simulink model "Host_IO_DataCapture"  (R2019b)
settings: Solver=FixedStepAuto  StartTime=0.0  StopTime=inf  FixedStep=(1/fpga_clk_rate)*4096  RelTol=1e-3  EnableMultiTasking=on
InitFcn:
  | model_init
values from neighbouring files (symbols this model uses):
  end_inc = round (((f1*2^N)/fpga_clk_rate)/VectorSamplingFactor)    [model_init.m]
  fpga_clk_rate = Fs/VectorSamplingFactor    (= 128000000)    [model_init.m]
  frameSize = 1536    [model_init.m]
  LFM_counter_inc = round((end_inc-start_inc)/PulseWidth_count)    [model_init.m]
  PulseWidth_count = pspshared.libiio.aximm.write(                    'IPAddress',IPAddr,                    'AddressOffset',hex2dec('13C'))    [SimplePulseGenerator_4x4_HDL_IQ_IIO_script.m]    (also in model_init.m = 640)
  RangeDelayTrigger_count = pspshared.libiio.aximm.write(                    'IPAddress',IPAddr,                    'AddressOffset',hex2dec('138'))    [SimplePulseGenerator_4x4_HDL_IQ_IIO_script.m]    (also in model_init.m = 1)
  start_inc = round (((f0*2^N)/fpga_clk_rate)/VectorSamplingFactor)    [model_init.m]
libraries: hdlsllib x16, simulink x2, psp_axi_iio_lib x1
Description:
  | 4x4 IQ ADC/DAC Data capture model for host PC
  | 
  | This model demonstrates capturing data from the FPGA for IQ mixer data. AXI4 register is used
  | to switch between different ADC channels and collect frames of data at every
  | time step of the simulation
  | 
  | The DAC is driven by an NCO. It's frequency is also adjustable from this model as well.
settings Model: Creator=darenlee  LastModifiedBy=ajtro
settings SolverCC: PositivePriorityOrder=on
settings DataIOCC: ReturnWorkspaceOutputs=off
settings OptimizationCC: DefaultParameterBehavior=Inlined  EnhancedBackFolding=on  PassReuseOutputArgsAs=Individual arguments  MaxStackSize=64  OptimizeBlockOrder=speed  DifferentSizesBufferReuse=on  OptimizationCustomize=off  EfficientTunableParamExpr=on
settings DebuggingCC: ParameterTunabilityLossMsg=error  PregeneratedLibrarySubsystemCodeDiagnostic=none  ArithmeticOperatorsInVariantConditions=warning
settings HardwareCC: ProdBitPerPointer=32  ProdBitPerSizeT=32  ProdBitPerPtrDiffT=32  ProdLargestAtomicInteger=Long  ProdLargestAtomicFloat=Double  ProdWordSize=32  ProdLongLongMode=on  ProdHWDeviceType=ARM Compatible->ARM Cortex
settings SFSimCC: SimUseLocalCustomCode=off  MATLABDynamicMemAlloc=off  CustomCodeUndefinedFunction=UseInterfaceOnly
settings RTWCC: SystemTargetFile=ert.tlc  TemplateMakefile=ert_default_tmf  GenerateReport=on  RTWUseLocalCustomCode=off  Toolchain=Linaro AArch32 Linux v6.3.1  IncludeHyperlinkInReport=on  LaunchReport=on  GenerateTraceInfo=on  GenerateTraceReport=on  GenerateTraceReportSl=on  GenerateTraceReportSf=on  GenerateTraceReportEml=on
settings CodeAppCC: ForceParamTrailComments=on  IgnoreCustomStorageClasses=off  OperatorAnnotations=on  SimulinkDataObjDesc=on  SFDataObjDesc=on  InsertBlockDesc=on
settings ERTTargetCC: ERTCustomFileTemplate=example_file_process.tlc

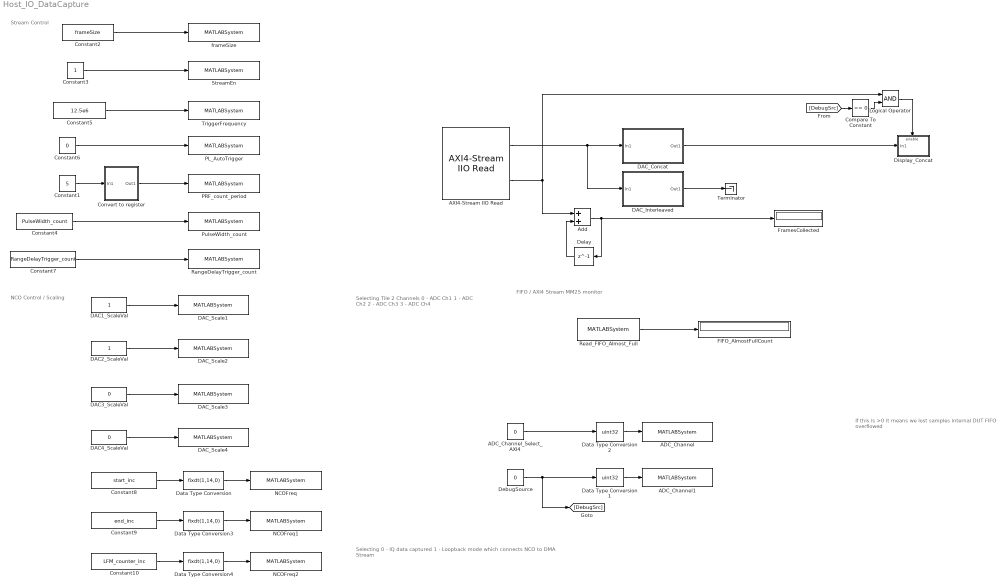
== system Host_IO_DataCapture ==
  note: Selecting Tile 2 Channels
      | 0 - ADC Ch1
      | 1 - ADC Ch2
      | 2 - ADC Ch3
      | 3 - ADC Ch4
  note: If this is >0 it means we lost samples
      | internal DUT FIFO overflowed
  note: FIFO / AXI4 Stream MM2S monitor
  note: Stream Control
  note: NCO Control / Scaling
  note: Selecting
      | 0 - IQ data captured
      | 1 - Loopback mode which connects NCO to DMA Stream
  ADC_Channel : MATLABSystem  System=pspshared.libiio.aximm.write  vectorModeEn=off  AddressOffsetSrc=Property  AddressOffset=hex2dec('114')  IPAddress=192.168.1.101  enIO=on  devName=mwipcore0:mmwr0
      settings: AttributesFormatString=%<AddressOffset>
      mask Type: pspshared.libiio.aximm.write
      mask Display:
      | color('white');
      | plot([100,100,100,100],[100,100,100,100]);
      | plot([0,0,0,0],[0,0,0,0]);
      | color('black');
      | text(50, 48,'AXI4 Register\nIIO Write', 'horizontalAlignment','center','verticalAlignment','middle');
      | color('blue');
      | text(95, 99, 'PSP', 'horizontalAlignment', 'right','verticalAlignment','top');
      | color('black');
      | port_label('input',1, 'Data')
  ADC_Channel1 : MATLABSystem  System=pspshared.libiio.aximm.write  vectorModeEn=off  AddressOffsetSrc=Property  AddressOffset=hex2dec('12C')  IPAddress=192.168.1.101  enIO=on  devName=mwipcore0:mmwr0
      settings: AttributesFormatString=%<AddressOffset>
      mask Type: pspshared.libiio.aximm.write
      mask Display:
      | color('white');
      | plot([100,100,100,100],[100,100,100,100]);
      | plot([0,0,0,0],[0,0,0,0]);
      | color('black');
      | text(50, 48,'AXI4 Register\nIIO Write', 'horizontalAlignment','center','verticalAlignment','middle');
      | color('blue');
      | text(95, 99, 'PSP', 'horizontalAlignment', 'right','verticalAlignment','top');
      | color('black');
      | port_label('input',1, 'Data')
  ADC_Channel_Select_AXI4 : Constant  Value=0  OutDataTypeStr=uint32  SampleTime=-1
  AXI4-Stream IIO Read : psp_axi_iio_lib/AXI4-Stream IIO Read  SamplesPerFrame=frameSize  DataType=ufix128  Timeout=0  IPAddress=192.168.1.101  enIO=on  devName=mwipcore0:s2mm0  IPResetMode=none  TLASTMode=auto  TLASTResetMode=prebuffer
      settings: SourceProductName=IIO AXI - PSP
  Add : Sum  AccumDataTypeStr=uint32  OutDataTypeStr=uint32
  Compare To Constant : simulink/Logic and Bit Operations/Compare To Constant  relop===  const=0  OutDataTypeStr=boolean
  Constant1 : Constant  Value=5
  Constant10 : Constant  Value=LFM_counter_inc  OutDataTypeStr=int32
  Constant2 : Constant  Value=frameSize  OutDataTypeStr=uint32  SampleTime=-1
  Constant3 : Constant  OutDataTypeStr=boolean  SampleTime=-1
  Constant4 : Constant  Value=PulseWidth_count  OutDataTypeStr=uint32
  Constant5 : Constant  Value=12.5e6  OutDataTypeStr=uint32  SampleTime=-1
  Constant6 : Constant  Value=0  OutDataTypeStr=boolean  SampleTime=-1
  Constant7 : Constant  Value=RangeDelayTrigger_count  OutDataTypeStr=uint32
  Constant8 : Constant  Value=start_inc  OutDataTypeStr=int32
  Constant9 : Constant  Value=end_inc  OutDataTypeStr=int32
  Convert to register : Subsystem
  DAC1_ScaleVal : Constant  OutDataTypeStr=fixdt(0,8,7)  SampleTime=-1
  DAC2_ScaleVal : Constant  OutDataTypeStr=fixdt(0,8,7)  SampleTime=-1
  DAC3_ScaleVal : Constant  Value=0  OutDataTypeStr=fixdt(0,8,7)  SampleTime=-1
  DAC4_ScaleVal : Constant  Value=0  OutDataTypeStr=fixdt(0,8,7)  SampleTime=-1
  DAC_Concat : Subsystem
  DAC_Interleaved : Subsystem
  DAC_Scale1 : MATLABSystem  System=pspshared.libiio.aximm.write  vectorModeEn=off  AddressOffsetSrc=Property  AddressOffset=hex2dec('11C')  IPAddress=192.168.1.101  enIO=on  devName=mwipcore0:mmwr0
      settings: AttributesFormatString=%<AddressOffset>
      mask Type: pspshared.libiio.aximm.write
      mask Display:
      | color('white');
      | plot([100,100,100,100],[100,100,100,100]);
      | plot([0,0,0,0],[0,0,0,0]);
      | color('black');
      | text(50, 48,'AXI4 Register\nIIO Write', 'horizontalAlignment','center','verticalAlignment','middle');
      | color('blue');
      | text(95, 99, 'PSP', 'horizontalAlignment', 'right','verticalAlignment','top');
      | color('black');
      | port_label('input',1, 'Data')
  DAC_Scale2 : MATLABSystem  System=pspshared.libiio.aximm.write  vectorModeEn=off  AddressOffsetSrc=Property  AddressOffset=hex2dec('120')  IPAddress=192.168.1.101  enIO=on  devName=mwipcore0:mmwr0
      settings: AttributesFormatString=%<AddressOffset>
      mask Type: pspshared.libiio.aximm.write
      mask Display:
      | color('white');
      | plot([100,100,100,100],[100,100,100,100]);
      | plot([0,0,0,0],[0,0,0,0]);
      | color('black');
      | text(50, 48,'AXI4 Register\nIIO Write', 'horizontalAlignment','center','verticalAlignment','middle');
      | color('blue');
      | text(95, 99, 'PSP', 'horizontalAlignment', 'right','verticalAlignment','top');
      | color('black');
      | port_label('input',1, 'Data')
  DAC_Scale3 : MATLABSystem  System=pspshared.libiio.aximm.write  vectorModeEn=off  AddressOffsetSrc=Property  AddressOffset=hex2dec('124')  IPAddress=192.168.1.101  enIO=on  devName=mwipcore0:mmwr0
      settings: AttributesFormatString=%<AddressOffset>
      mask Type: pspshared.libiio.aximm.write
      mask Display:
      | color('white');
      | plot([100,100,100,100],[100,100,100,100]);
      | plot([0,0,0,0],[0,0,0,0]);
      | color('black');
      | text(50, 48,'AXI4 Register\nIIO Write', 'horizontalAlignment','center','verticalAlignment','middle');
      | color('blue');
      | text(95, 99, 'PSP', 'horizontalAlignment', 'right','verticalAlignment','top');
      | color('black');
      | port_label('input',1, 'Data')
  DAC_Scale4 : MATLABSystem  System=pspshared.libiio.aximm.write  vectorModeEn=off  AddressOffsetSrc=Property  AddressOffset=hex2dec('128')  IPAddress=192.168.1.101  enIO=on  devName=mwipcore0:mmwr0
      settings: AttributesFormatString=%<AddressOffset>
      mask Type: pspshared.libiio.aximm.write
      mask Display:
      | color('white');
      | plot([100,100,100,100],[100,100,100,100]);
      | plot([0,0,0,0],[0,0,0,0]);
      | color('black');
      | text(50, 48,'AXI4 Register\nIIO Write', 'horizontalAlignment','center','verticalAlignment','middle');
      | color('blue');
      | text(95, 99, 'PSP', 'horizontalAlignment', 'right','verticalAlignment','top');
      | color('black');
      | port_label('input',1, 'Data')
  Data Type Conversion : DataTypeConversion  OutMin=8191  OutMax=8191  OutDataTypeStr=fixdt(1,14,0)
  Data Type Conversion1 : DataTypeConversion  OutDataTypeStr=uint32
  Data Type Conversion2 : DataTypeConversion  OutDataTypeStr=uint32
  Data Type Conversion3 : DataTypeConversion  OutMin=8191  OutMax=8191  OutDataTypeStr=fixdt(1,14,0)
  Data Type Conversion4 : DataTypeConversion  OutMin=8191  OutMax=8191  OutDataTypeStr=fixdt(1,14,0)
  DebugSource : Constant  Value=0  OutDataTypeStr=uint32  SampleTime=-1
  Delay : Delay  DelayLength=1
  Display_Concat : Subsystem
  FIFO_AlmostFullCount : Display
  FramesCollected : Display
  Logical Operator : Logic  AllPortsSameDT=off  OutDataTypeStr=boolean
  NCOFreq : MATLABSystem  System=pspshared.libiio.aximm.write  vectorModeEn=off  AddressOffsetSrc=Property  AddressOffset=hex2dec('118')  IPAddress=192.168.1.101  enIO=on  devName=mwipcore0:mmwr0
      settings: AttributesFormatString=%<AddressOffset>
      mask Type: pspshared.libiio.aximm.write
      mask Display:
      | color('white');
      | plot([100,100,100,100],[100,100,100,100]);
      | plot([0,0,0,0],[0,0,0,0]);
      | color('black');
      | text(50, 48,'AXI4 Register\nIIO Write', 'horizontalAlignment','center','verticalAlignment','middle');
      | color('blue');
      | text(95, 99, 'PSP', 'horizontalAlignment', 'right','verticalAlignment','top');
      | color('black');
      | port_label('input',1, 'Data')
  NCOFreq1 : MATLABSystem  System=pspshared.libiio.aximm.write  vectorModeEn=off  AddressOffsetSrc=Property  AddressOffset=hex2dec('100')  IPAddress=192.168.1.101  enIO=on  devName=mwipcore0:mmwr0
      settings: AttributesFormatString=%<AddressOffset>
      mask Type: pspshared.libiio.aximm.write
      mask Display:
      | color('white');
      | plot([100,100,100,100],[100,100,100,100]);
      | plot([0,0,0,0],[0,0,0,0]);
      | color('black');
      | text(50, 48,'AXI4 Register\nIIO Write', 'horizontalAlignment','center','verticalAlignment','middle');
      | color('blue');
      | text(95, 99, 'PSP', 'horizontalAlignment', 'right','verticalAlignment','top');
      | color('black');
      | port_label('input',1, 'Data')
  NCOFreq2 : MATLABSystem  System=pspshared.libiio.aximm.write  vectorModeEn=off  AddressOffsetSrc=Property  AddressOffset=hex2dec('140')  IPAddress=192.168.1.101  enIO=on  devName=mwipcore0:mmwr0
      settings: AttributesFormatString=%<AddressOffset>
      mask Type: pspshared.libiio.aximm.write
      mask Display:
      | color('white');
      | plot([100,100,100,100],[100,100,100,100]);
      | plot([0,0,0,0],[0,0,0,0]);
      | color('black');
      | text(50, 48,'AXI4 Register\nIIO Write', 'horizontalAlignment','center','verticalAlignment','middle');
      | color('blue');
      | text(95, 99, 'PSP', 'horizontalAlignment', 'right','verticalAlignment','top');
      | color('black');
      | port_label('input',1, 'Data')
  PL_AutoTrigger : MATLABSystem  System=pspshared.libiio.aximm.write  vectorModeEn=off  AddressOffsetSrc=Property  AddressOffset=hex2dec('110')  IPAddress=192.168.1.101  enIO=on  devName=mwipcore0:mmwr0
      settings: AttributesFormatString=%<AddressOffset>
      mask Type: pspshared.libiio.aximm.write
      mask Display:
      | color('white');
      | plot([100,100,100,100],[100,100,100,100]);
      | plot([0,0,0,0],[0,0,0,0]);
      | color('black');
      | text(50, 48,'AXI4 Register\nIIO Write', 'horizontalAlignment','center','verticalAlignment','middle');
      | color('blue');
      | text(95, 99, 'PSP', 'horizontalAlignment', 'right','verticalAlignment','top');
      | color('black');
      | port_label('input',1, 'Data')
  PRF_count_period : MATLABSystem  System=pspshared.libiio.aximm.write  vectorModeEn=off  AddressOffsetSrc=Property  AddressOffset=hex2dec('130')  IPAddress=192.168.1.101  enIO=on  devName=mwipcore0:mmwr0
      settings: AttributesFormatString=%<AddressOffset>
      mask Type: pspshared.libiio.aximm.write
      mask Display:
      | color('white');
      | plot([100,100,100,100],[100,100,100,100]);
      | plot([0,0,0,0],[0,0,0,0]);
      | color('black');
      | text(50, 48,'AXI4 Register\nIIO Write', 'horizontalAlignment','center','verticalAlignment','middle');
      | color('blue');
      | text(95, 99, 'PSP', 'horizontalAlignment', 'right','verticalAlignment','top');
      | color('black');
      | port_label('input',1, 'Data')
  PulseWidth_count : MATLABSystem  System=pspshared.libiio.aximm.write  vectorModeEn=off  AddressOffsetSrc=Property  AddressOffset=hex2dec('13C')  IPAddress=192.168.1.101  enIO=on  devName=mwipcore0:mmwr0
      settings: AttributesFormatString=%<AddressOffset>
      mask Type: pspshared.libiio.aximm.write
      mask Display:
      | color('white');
      | plot([100,100,100,100],[100,100,100,100]);
      | plot([0,0,0,0],[0,0,0,0]);
      | color('black');
      | text(50, 48,'AXI4 Register\nIIO Write', 'horizontalAlignment','center','verticalAlignment','middle');
      | color('blue');
      | text(95, 99, 'PSP', 'horizontalAlignment', 'right','verticalAlignment','top');
      | color('black');
      | port_label('input',1, 'Data')
  RangeDelayTrigger_count : MATLABSystem  System=pspshared.libiio.aximm.write  vectorModeEn=off  AddressOffsetSrc=Property  AddressOffset=hex2dec('138')  IPAddress=192.168.1.101  enIO=on  devName=mwipcore0:mmwr0
      settings: AttributesFormatString=%<AddressOffset>
      mask Type: pspshared.libiio.aximm.write
      mask Display:
      | color('white');
      | plot([100,100,100,100],[100,100,100,100]);
      | plot([0,0,0,0],[0,0,0,0]);
      | color('black');
      | text(50, 48,'AXI4 Register\nIIO Write', 'horizontalAlignment','center','verticalAlignment','middle');
      | color('blue');
      | text(95, 99, 'PSP', 'horizontalAlignment', 'right','verticalAlignment','top');
      | color('black');
      | port_label('input',1, 'Data')
  Read_FIFO_Almost_Full : MATLABSystem  System=pspshared.libiio.aximm.read  DataType=uint32  vectorModeEn=off  outputVectorLength=2  AddressOffsetSrc=Property  AddressOffset=hex2dec('134')  IPAddress=192.168.1.101  enIO=on  FixedPointDataTypeStr=fixdt(0,14,0)  devName=mwipcore0:mmrd0
      settings: AttributesFormatString=%<AddressOffset>
      mask Type: pspshared.libiio.aximm.read
      mask Display:
      | color('white');
      | plot([100,100,100,100],[100,100,100,100]);
      | plot([0,0,0,0],[0,0,0,0]);
      | color('black');
      | text(50, 48,'AXI4 Register\nIIO Read', 'horizontalAlignment','center','verticalAlignment','middle');
      | color('blue');
      | text(95, 99, 'PSP', 'horizontalAlignment', 'right','verticalAlignment','top');
      | color('black');
      | port_label('output',1, 'Data')
  StreamEn : MATLABSystem  System=pspshared.libiio.aximm.write  vectorModeEn=off  AddressOffsetSrc=Property  AddressOffset=hex2dec('108')  IPAddress=192.168.1.101  enIO=on  devName=mwipcore0:mmwr0
      settings: AttributesFormatString=%<AddressOffset>
      mask Type: pspshared.libiio.aximm.write
      mask Display:
      | color('white');
      | plot([100,100,100,100],[100,100,100,100]);
      | plot([0,0,0,0],[0,0,0,0]);
      | color('black');
      | text(50, 48,'AXI4 Register\nIIO Write', 'horizontalAlignment','center','verticalAlignment','middle');
      | color('blue');
      | text(95, 99, 'PSP', 'horizontalAlignment', 'right','verticalAlignment','top');
      | color('black');
      | port_label('input',1, 'Data')
  Terminator : Terminator
  TriggerFrequency : MATLABSystem  System=pspshared.libiio.aximm.write  vectorModeEn=off  AddressOffsetSrc=Property  AddressOffset=hex2dec('10C')  IPAddress=192.168.1.101  enIO=on  devName=mwipcore0:mmwr0
      settings: AttributesFormatString=%<AddressOffset>
      mask Type: pspshared.libiio.aximm.write
      mask Display:
      | color('white');
      | plot([100,100,100,100],[100,100,100,100]);
      | plot([0,0,0,0],[0,0,0,0]);
      | color('black');
      | text(50, 48,'AXI4 Register\nIIO Write', 'horizontalAlignment','center','verticalAlignment','middle');
      | color('blue');
      | text(95, 99, 'PSP', 'horizontalAlignment', 'right','verticalAlignment','top');
      | color('black');
      | port_label('input',1, 'Data')
  frameSize : MATLABSystem  System=pspshared.libiio.aximm.write  vectorModeEn=off  AddressOffsetSrc=Property  AddressOffset=hex2dec('104')  IPAddress=192.168.1.101  enIO=on  devName=mwipcore0:mmwr0
      settings: AttributesFormatString=%<AddressOffset>
      mask Type: pspshared.libiio.aximm.write
      mask Display:
      | color('white');
      | plot([100,100,100,100],[100,100,100,100]);
      | plot([0,0,0,0],[0,0,0,0]);
      | color('black');
      | text(50, 48,'AXI4 Register\nIIO Write', 'horizontalAlignment','center','verticalAlignment','middle');
      | color('blue');
      | text(95, 99, 'PSP', 'horizontalAlignment', 'right','verticalAlignment','top');
      | color('black');
      | port_label('input',1, 'Data')
  wires:
  AXI4-Stream IIO Read/2 -> Add/1, Logical Operator/1
  Constant2/1 -> frameSize/1
  Constant3/1 -> StreamEn/1
  Delay/1 -> Add/2
  Add/1 -> Delay/1, FramesCollected/1
  Data Type Conversion/1 -> NCOFreq/1
  DAC1_ScaleVal/1 -> DAC_Scale1/1
  DAC2_ScaleVal/1 -> DAC_Scale2/1
  DAC3_ScaleVal/1 -> DAC_Scale3/1
  DAC4_ScaleVal/1 -> DAC_Scale4/1
  Constant8/1 -> Data Type Conversion/1
  Constant5/1 -> TriggerFrequency/1
  Constant6/1 -> PL_AutoTrigger/1
  Read_FIFO_Almost_Full/1 -> FIFO_AlmostFullCount/1
  Data Type Conversion2/1 -> ADC_Channel/1
  ADC_Channel_Select_AXI4/1 -> Data Type Conversion2/1
  Data Type Conversion1/1 -> ADC_Channel1/1
  AXI4-Stream IIO Read/1 -> DAC_Interleaved/1(In1), DAC_Concat/1(In1)
  DAC_Concat/1(Out1) -> Display_Concat/1(In1)
  DAC_Interleaved/1(Out1) -> Terminator/1
  DebugSource/1 -> [DebugSrc], Data Type Conversion1/1
  [DebugSrc] -> Compare To Constant/1
  Compare To Constant/1 -> Logical Operator/2
  Logical Operator/1 -> Display_Concat/Enable
  Constant1/1 -> Convert to register/1(In1)
  Convert to register/1(Out1) -> PRF_count_period/1
  Constant4/1 -> PulseWidth_count/1
  Constant7/1 -> RangeDelayTrigger_count/1
  Constant9/1 -> Data Type Conversion3/1
  Data Type Conversion3/1 -> NCOFreq1/1
  Data Type Conversion4/1 -> NCOFreq2/1
  Constant10/1 -> Data Type Conversion4/1

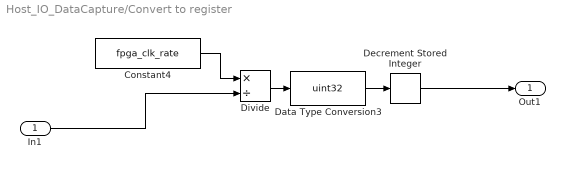
== system Host_IO_DataCapture/Convert to register ==
  In1 : Inport
  Constant4 : Constant  Value=fpga_clk_rate
  Data Type Conversion3 : DataTypeConversion  OutDataTypeStr=uint32
  Decrement Stored Integer : simulink/Additional Math & Discrete/Additional Math: Increment - Decrement/Decrement Stored Integer
      settings: SourceProductName=Simulink  SourceProductBaseCode=SL
  Divide : Product  Inputs=*/
  Out1 : Outport
  wires:
  Data Type Conversion3/1 -> Decrement Stored Integer/1
  Divide/1 -> Data Type Conversion3/1
  Decrement Stored Integer/1 -> Out1/1
  Constant4/1 -> Divide/1
  In1/1 -> Divide/2

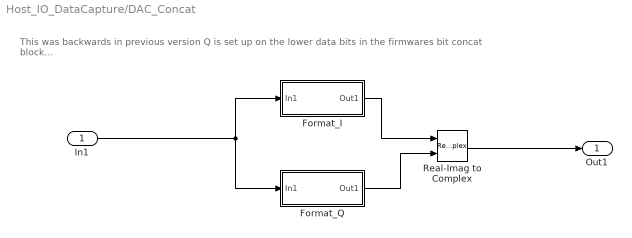
== system Host_IO_DataCapture/DAC_Concat ==
  note: This was backwards in previous version Q is set up on the lower data bits in the firmwares bit concat block...
  In1 : Inport
  Format_I : Subsystem
  Format_Q : Subsystem
  Real-Imag to Complex : RealImagToComplex
  Out1 : Outport  VectorParamsAs1DForOutWhenUnconnected=off
  wires:
  Format_I/1(Out1) -> Real-Imag to Complex/1
  In1/1 -> Format_I/1(In1), Format_Q/1(In1)
  Real-Imag to Complex/1 -> Out1/1
  Format_Q/1(Out1) -> Real-Imag to Complex/2

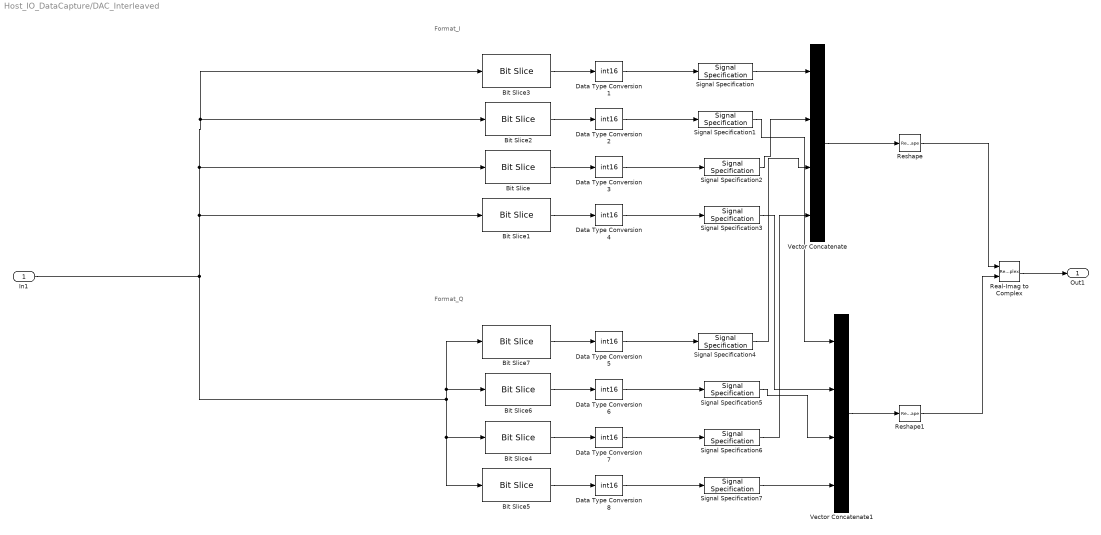
== system Host_IO_DataCapture/DAC_Interleaved ==
  note: Format_Q
  note: Format_I
  In1 : Inport
  Bit Slice : hdlsllib/Logic and Bit Operations/Bit Slice  lidx=47  ridx=32
  Bit Slice1 : hdlsllib/Logic and Bit Operations/Bit Slice  lidx=63  ridx=48
  Bit Slice2 : hdlsllib/Logic and Bit Operations/Bit Slice  lidx=31  ridx=16
  Bit Slice3 : hdlsllib/Logic and Bit Operations/Bit Slice  lidx=15  ridx=0
  Bit Slice4 : hdlsllib/Logic and Bit Operations/Bit Slice  lidx=111  ridx=96
  Bit Slice5 : hdlsllib/Logic and Bit Operations/Bit Slice  lidx=127  ridx=112
  Bit Slice6 : hdlsllib/Logic and Bit Operations/Bit Slice  lidx=95  ridx=80
  Bit Slice7 : hdlsllib/Logic and Bit Operations/Bit Slice  lidx=79  ridx=64
  Data Type Conversion{1..8} (8 alike) : DataTypeConversion  OutDataTypeStr=int16  ConvertRealWorld=Stored Integer (SI)
  Real-Imag to Complex : RealImagToComplex
  Reshape : Reshape
  Reshape1 : Reshape
  Signal Specification{,1..7} (8 alike) : SignalSpecification  Dimensions=[1 frameSize]
  Vector Concatenate : Concatenate  NumInputs=4  Mode=Multidimensional array
  Vector Concatenate1 : Concatenate  NumInputs=4  Mode=Multidimensional array
  Out1 : Outport  VectorParamsAs1DForOutWhenUnconnected=off
  wires:
  Reshape/1 -> Real-Imag to Complex/1
  Real-Imag to Complex/1 -> Out1/1
  Reshape1/1 -> Real-Imag to Complex/2
  Data Type Conversion3/1 -> Signal Specification2/1
  Bit Slice2/1 -> Data Type Conversion2/1
  Data Type Conversion1/1 -> Signal Specification/1
  Data Type Conversion4/1 -> Signal Specification3/1
  Data Type Conversion2/1 -> Signal Specification1/1
  Bit Slice/1 -> Data Type Conversion3/1
  Bit Slice1/1 -> Data Type Conversion4/1
  Signal Specification/1 -> Vector Concatenate/1
  Vector Concatenate/1 -> Reshape/1
  Bit Slice3/1 -> Data Type Conversion1/1
  Data Type Conversion7/1 -> Signal Specification6/1
  Bit Slice6/1 -> Data Type Conversion6/1
  Data Type Conversion5/1 -> Signal Specification4/1
  Data Type Conversion8/1 -> Signal Specification7/1
  Data Type Conversion6/1 -> Signal Specification5/1
  Bit Slice4/1 -> Data Type Conversion7/1
  Bit Slice5/1 -> Data Type Conversion8/1
  Vector Concatenate1/1 -> Reshape1/1
  Bit Slice7/1 -> Data Type Conversion5/1
  In1/1 -> Bit Slice5/1, Bit Slice4/1, Bit Slice7/1, Bit Slice6/1, Bit Slice3/1, Bit Slice2/1, Bit Slice/1, Bit Slice1/1
  Signal Specification2/1 -> Vector Concatenate/2
  Signal Specification4/1 -> Vector Concatenate/3
  Signal Specification6/1 -> Vector Concatenate/4
  Signal Specification1/1 -> Vector Concatenate1/1
  Signal Specification3/1 -> Vector Concatenate1/2
  Signal Specification5/1 -> Vector Concatenate1/3
  Signal Specification7/1 -> Vector Concatenate1/4

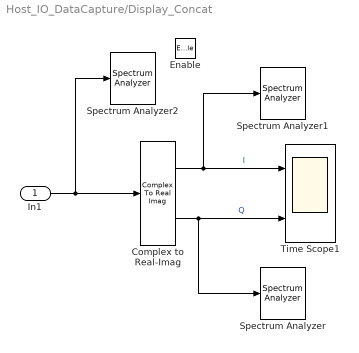
== system Host_IO_DataCapture/Display_Concat ==
  In1 : Inport
  Enable : EnablePort
  Complex to Real-Imag : ComplexToRealImag
  Spectrum Analyzer : SpectrumAnalyzer
  Spectrum Analyzer1 : SpectrumAnalyzer
  Spectrum Analyzer2 : SpectrumAnalyzer
  Time Scope1 : Scope  NumInputPorts=2
  wires:
  In1/1 -> Spectrum Analyzer2/1, Complex to Real-Imag/1
  Complex to Real-Imag/1 -> Spectrum Analyzer1/1, Time Scope1/1  "I"
  Complex to Real-Imag/2 -> Spectrum Analyzer/1, Time Scope1/2  "Q"

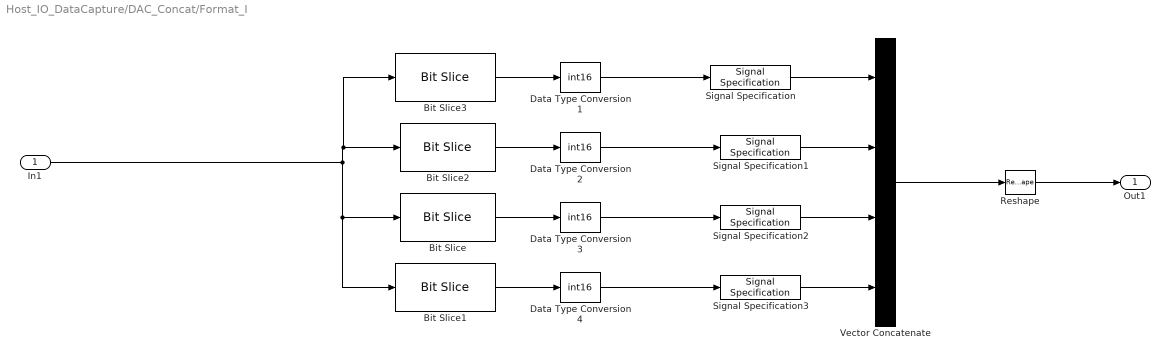
== system Host_IO_DataCapture/DAC_Concat/Format_I ==
  In1 : Inport
  Bit Slice : hdlsllib/Logic and Bit Operations/Bit Slice  lidx=111  ridx=96
  Bit Slice1 : hdlsllib/Logic and Bit Operations/Bit Slice  lidx=127  ridx=112
  Bit Slice2 : hdlsllib/Logic and Bit Operations/Bit Slice  lidx=95  ridx=80
  Bit Slice3 : hdlsllib/Logic and Bit Operations/Bit Slice  lidx=79  ridx=64
  Data Type Conversion{1..4} (4 alike) : DataTypeConversion  OutDataTypeStr=int16  ConvertRealWorld=Stored Integer (SI)
  Reshape : Reshape
  Signal Specification{,1..3} (4 alike) : SignalSpecification  Dimensions=[1 frameSize]
  Vector Concatenate : Concatenate  NumInputs=4  Mode=Multidimensional array
  Out1 : Outport  VectorParamsAs1DForOutWhenUnconnected=off
  wires:
  In1/1 -> Bit Slice1/1, Bit Slice/1, Bit Slice3/1, Bit Slice2/1
  Bit Slice3/1 -> Data Type Conversion1/1
  Vector Concatenate/1 -> Reshape/1
  Signal Specification3/1 -> Vector Concatenate/4
  Signal Specification2/1 -> Vector Concatenate/3
  Signal Specification/1 -> Vector Concatenate/1
  Bit Slice1/1 -> Data Type Conversion4/1
  Bit Slice/1 -> Data Type Conversion3/1
  Signal Specification1/1 -> Vector Concatenate/2
  Reshape/1 -> Out1/1
  Data Type Conversion2/1 -> Signal Specification1/1
  Data Type Conversion4/1 -> Signal Specification3/1
  Data Type Conversion1/1 -> Signal Specification/1
  Bit Slice2/1 -> Data Type Conversion2/1
  Data Type Conversion3/1 -> Signal Specification2/1

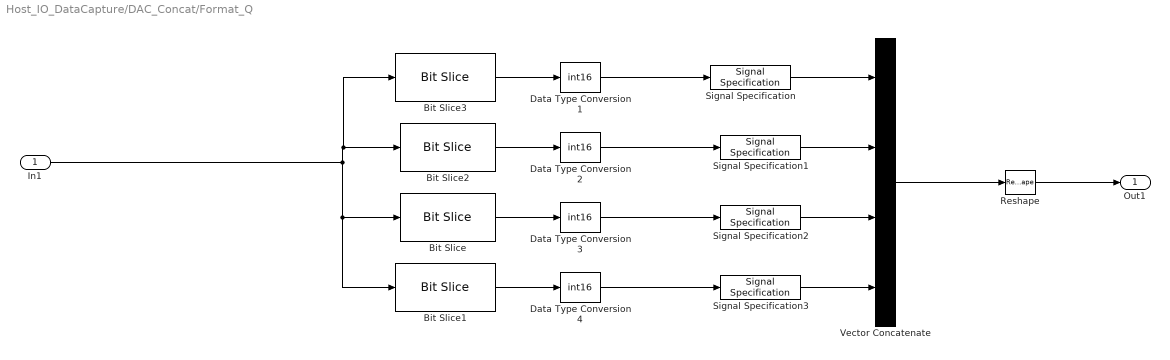
== system Host_IO_DataCapture/DAC_Concat/Format_Q ==
  In1 : Inport
  Bit Slice : hdlsllib/Logic and Bit Operations/Bit Slice  lidx=47  ridx=32
  Bit Slice1 : hdlsllib/Logic and Bit Operations/Bit Slice  lidx=63  ridx=48
  Bit Slice2 : hdlsllib/Logic and Bit Operations/Bit Slice  lidx=31  ridx=16
  Bit Slice3 : hdlsllib/Logic and Bit Operations/Bit Slice  lidx=15  ridx=0
  Data Type Conversion{1..4} (4 alike) : DataTypeConversion  OutDataTypeStr=int16  ConvertRealWorld=Stored Integer (SI)
  Reshape : Reshape
  Signal Specification{,1..3} (4 alike) : SignalSpecification  Dimensions=[1 frameSize]
  Vector Concatenate : Concatenate  NumInputs=4  Mode=Multidimensional array
  Out1 : Outport  VectorParamsAs1DForOutWhenUnconnected=off
  wires:
  In1/1 -> Bit Slice1/1, Bit Slice/1, Bit Slice3/1, Bit Slice2/1
  Bit Slice3/1 -> Data Type Conversion1/1
  Vector Concatenate/1 -> Reshape/1
  Signal Specification3/1 -> Vector Concatenate/4
  Signal Specification2/1 -> Vector Concatenate/3
  Signal Specification/1 -> Vector Concatenate/1
  Bit Slice1/1 -> Data Type Conversion4/1
  Bit Slice/1 -> Data Type Conversion3/1
  Signal Specification1/1 -> Vector Concatenate/2
  Reshape/1 -> Out1/1
  Data Type Conversion2/1 -> Signal Specification1/1
  Data Type Conversion4/1 -> Signal Specification3/1
  Data Type Conversion1/1 -> Signal Specification/1
  Bit Slice2/1 -> Data Type Conversion2/1
  Data Type Conversion3/1 -> Signal Specification2/1
